simulink library "CIFFT"  (R2022b)
settings: Solver=VariableStepAuto  StartTime=0.0  StopTime=10.0  RelTol=1e-3
settings Model: Creator=pk47312  LastModifiedBy=kl13806
settings SolverCC: AlgebraicLoopSolver=TrustRegion
settings DebuggingCC: UnconnectedInputMsg=warning  UnconnectedOutputMsg=warning  UnconnectedLineMsg=warning  SFMachineParentedDataDiag=warning  ArithmeticOperatorsInVariantConditions=warning
settings ModelReferenceCC: EnableRefExpFcnMdlSchedulingChecks=on
settings SFSimCC: CustomCodeUndefinedFunction=UseInterfaceOnly
settings RTWCC: DLArmComputeVersion=19.05

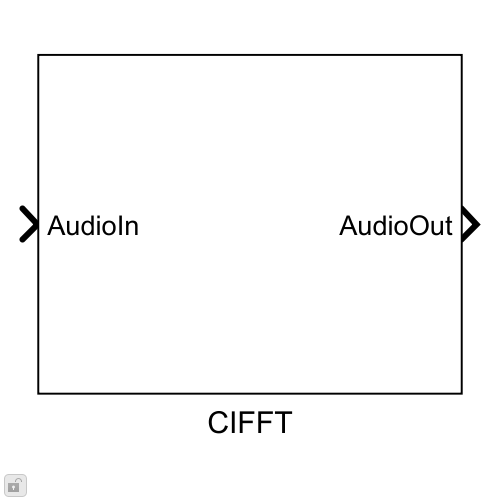
[thumbnail: Simulink's stored preview of the top-level diagram]
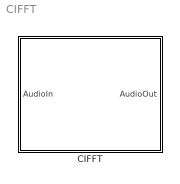
== system CIFFT ==
  CIFFT : Subsystem  mask(Complex IFFT){fftSize=256}
      mask prompts: fftSize "FFT size:"
      mask help: FFT size must power of 2, no more than 256 and no less than 8.
      mask init:
      | defaultTwiddleSize = 128; % this is equal to half of the max supported fft size
      | twiddleStride = 2 * defaultTwiddleSize / fftSize;
      | 
      | supportSizes = [8, 16, 32, 64, 128, 256];
      | if ~ismember(fftSize, supportSizes)
      |     error('FFT size must power of 2, no more than 256 and no less than 8.');
      | end

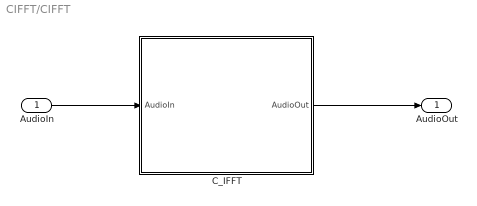
== system CIFFT/CIFFT ==
  AudioIn : Inport
  C_IFFT : MATLAB Function  TreatAsAtomicUnit=on
  AudioOut : Outport  VectorParamsAs1DForOutWhenUnconnected=off
  wires:
  AudioIn/1 -> C_IFFT/1(AudioIn)
  C_IFFT/1(AudioOut) -> AudioOut/1

== matlab function CIFFT/C_IFFT ==
  data fftSize settings: description=Length of the FFT
  data: AudioIn input; AudioOut output; fftSize parameter; twiddleStride parameter
function AudioOut = c_ifft(AudioIn, fftSize, twiddleStride)
    % Cast input to complex if needed
    if (isreal(AudioIn))
        input = complex(AudioIn);
    else 
        input = AudioIn;
    end
    
    % nullcopy copies type, size, and complexity of input to output
    AudioOut = coder.nullcopy(input);
    [frameSize, numChannels] = size(AudioIn);
    
    % Set correct data types
    fftSize = uint32(fftSize);
    numChannels = uint32(numChannels);
    twiddleStride = int32(twiddleStride);
    
    % Create temp buffer to store the temporary result generared by FFT
    persistent temp;
    if(isempty(temp))
        temp = complex(single(zeros(frameSize, numChannels)));
    end
    % Invoke cifft_f function
    AudioOut = cifft_f(input, temp, fftSize, numChannels, twiddleStride);
end

function y = cifft_f(AudioIn, temp1, fft_size, num_channel, twiddle_stride)
   % If code gen'ing, generate a warning if this is not replaced with
   % cifft_f
   coder.replace('-warnifnoreplacement');
   y = ifft(AudioIn);
end
